simulink model "SSR_FIR"  (R2025a)
settings: Solver=VariableStepAuto  StartTime=0.0  StopTime=1000  RelTol=1e-3
InitFcn:
  | SSR=8;
  | TAPS=64;
  | Ts=1/SSR;
  | FCOEFF = fir1(TAPS-1,0.25);
undefined symbols (not defined in the file or in its folder): S, vsva2197, xcvc1902
libraries: hdlSSR x12, hdlBasic x6, hdlUtilities x3, dspsrcs4 x1, dspobslib x1, vmcUtilities x1
settings Model: Creator=catalinb  LastModifiedBy=robg
settings SolverCC: AlgebraicLoopSolver=TrustRegion
settings DebuggingCC: UnconnectedInputMsg=warning  UnconnectedOutputMsg=warning  UnconnectedLineMsg=warning
settings ModelReferenceCC: EnableRefExpFcnMdlSchedulingChecks=on
settings RTWCC: GPUComputeCapability=3.5  DLArmComputeVersion=19.05

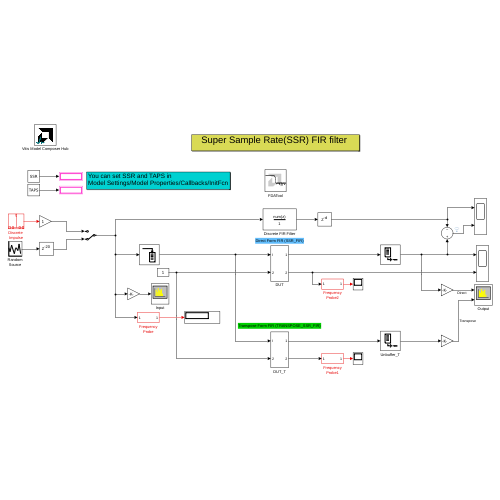
[thumbnail: Simulink's stored preview of the top-level diagram]
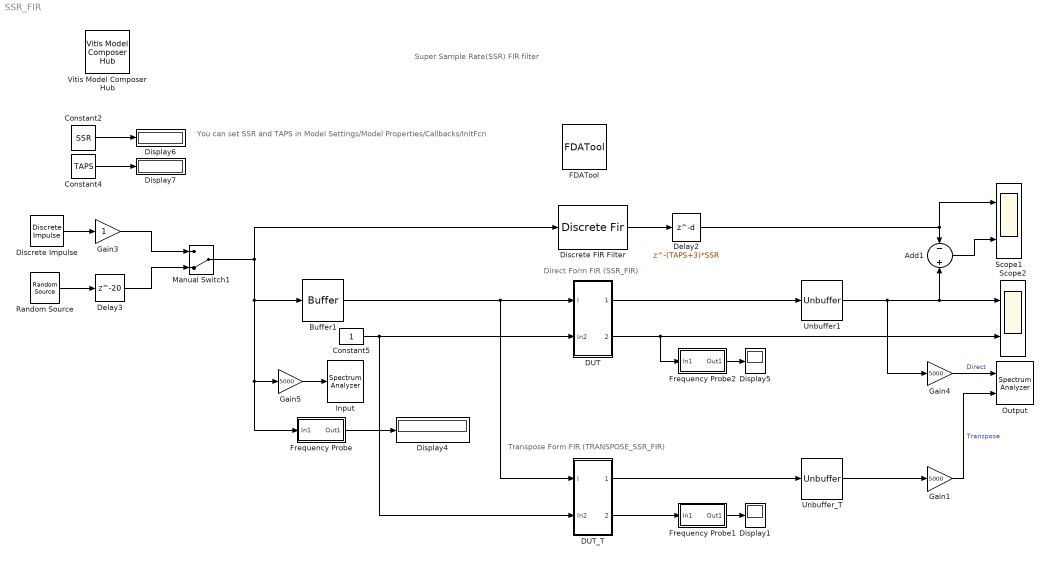
== system SSR_FIR ==
  note: You can set SSR and TAPS in
      | Model Settings/Model Properties/Callbacks/InitFcn
  note: Super Sample Rate(SSR) FIR filter
  note: Direct Form FIR (SSR_FIR)
  note: Transpose Form FIR (TRANSPOSE_SSR_FIR)
  Add1 : Sum  Inputs=-|+
  Buffer1 : Buffer  N=SSR  OutputFrames=off
  Constant2 : Constant  Value=SSR
  Constant4 : Constant  Value=TAPS
  Constant5 : Constant  SampleTime=-1
  DUT : Subsystem
  DUT_T : Subsystem
  Delay2 : Delay  DelayLength=(TAPS+3)*SSR
  Delay3 : Delay  DelayLength=20
  Discrete Impulse : dspsrcs4/Discrete  Impulse  SFcnStateName=COUNT  Delay=19  SampleTime=Ts  FrameSample=1  OutputFrames=off  dataType=double  isSigned=on  wordLen=16  udDataType=sfix(16)  fracBitsMode=Best precision  numFracBits=15  OutDataTypeStr=double  LastOutDataTypeStr=double
      settings: SFcnIsStateOwnerBlock=on
  Discrete FIR Filter : DiscreteFir  Coefficients=FCOEFF  InputProcessing=Columns as channels (frame based)
  Display{1,4..7} (5 alike) : Display
  FDATool : hdlUtilities/FDATool  block_type=fdatool
      settings: infoedit=FDATool
  Frequency Probe : Subsystem
  Frequency Probe1 : Subsystem
  Frequency Probe2 : Subsystem
  Gain1 : Gain  Gain=5000
  Gain3 : Gain
  Gain4 : Gain  Gain=5000
  Gain5 : Gain  Gain=5000
  Input : SpectrumAnalyzer  WindowPosition=[892.000000,252.000000,808.000000,450.000000,]  ScopeFrameLocation=window  SampleRate=5  AxesScaling=Manual  Span=8  StartFrequency=-4  StopFrequency=4  AveragingMethod=Exponential  YLimits=[35.8582 80.9757]  ChannelNames="[\"\"]"  AllowFFTLengthLessThanSamplesPerUpdate=on  DefaultConfigurationName=spbscopes.SpectrumAnalyzerBlockCfg
  Manual Switch1 : ManualSwitch  CurrentSetting=0
  Output : SpectrumAnalyzer  NumInputPorts=2  WindowPosition=[131.000000,278.000000,802.000000,452.000000,]  ScopeFrameLocation=window  SampleRate=5  AxesScaling=Manual  Span=8  StartFrequency=-4  StopFrequency=4  AveragingMethod=Exponential  YLimits=[-125.0298,37.1965]  ShowLegend=on  ChannelNames="[\"\"]"  AllowFFTLengthLessThanSamplesPerUpdate=on  DefaultConfigurationName=spbscopes.SpectrumAnalyzerBlockCfg
  Random Source : dspobslib/Random Source  SrcType=Uniform  NormMethod=Ziggurat  CltLength=12  MinVal=-1  MaxVal=1  MeanVal=0  VarVal=1  RepMode=Not repeatable  rawSeed=1  IsInherit=off  SampMode=Discrete  SampTime=Ts  SampFrame=1  DataType=Double  OutComplex=Real  OutputFrames=off
  Scope1 : Scope  NumInputPorts=2
      settings: ActiveDisplayYMinimum=-1.4468  ActiveDisplayYMaximum=1.4114  DataLoggingVariableName=ScopeData2
  Scope2 : Scope  NumInputPorts=2
      settings: ActiveDisplayYMinimum=-0.75312  ActiveDisplayYMaximum=0.71474
  Unbuffer1 : Unbuffer
  Unbuffer_T : Unbuffer
  Vitis Model Composer Hub : vmcUtilities/Vitis Model Composer Hub  Tag=genX  CodeGeneration=off  SubsystemName=DUT  BlockHierPath=SSR_FIR/DUT  CompilationType=HDLCompilation  SubsystemType=HDLNode  ExportTypeV2=IP Catalog  StartColumn=1  NumberOfColumns=1  TargetDirectory=./netlist  exportDesign=on  analyzeDesign=off  validateDesignOnHw=off  ExportType=AI Engines  IpVendor=xilinx.com  IpLibrary=hls  IpVersion=1.0  IpHWLanguage=Verilog  AieCompilerOptions={}  AieSimulatorOptions={}  CreateTestbench=off  TestbenchStackSize=10  RunRtlSim=off  RunCSim=off  RunAieSim=off  enableSimulationTimeout=on  enableGraphIterations=on  AieSimTimeout=50000  AieGraphIterations=-1  RunAieSimProfiling=off  LaunchVitisAnalyzer=off  PlotOutput=off  RunX86Sim=off  X86SimTimeout=10  GenHwImage=off  GenLibadfXo=on  GenHwValidationCode=off  PlatformType=Not Specified  HwSystemType=Baremetal  HwValidationTarget=hw  ProjDevice=xcvc1902-vsva2197-1LP-e-S  ProjDevicePart=xcvc1902-vsva2197-1LP-e-S  AIEType=AIE  SamplePeriod=-1  ClockFrequency=200  DataPathParallelism=1  xilinxfamily=versalaicore  part=xcvc1902  speed=-1LP-e-S  package=vsva2197  directory=./netlist/ip/DUT/src  testbench=off  incr_netlist=off  synthesis_tool=Vivado  clock_wrapper=Clock Enables  dbl_ovrd=According to Block Masks  dcm_input_clock_period=10  sysclk_period=10  simulink_period=1  eval_field=0  IPInfoJsonString="{\"DUTSubsystemName\":\"DUT\",\"HDLSubsystem\":{\"SubsystemName\":\"DUT\",\"IPName\":\"SSR_fir\",\"IPLibrary\":\"VMC\",\"IPVendor\":\"User Company\",\"IPVersion\":\"1.0\",\"TargetDirectory\":\"./netlist\",\"SubsystemDir\":\"./netlist/ip/DUT\",\"FreqHz\":\"100000000\"},\"SubsystemTag\":\"HDLNode\"}"  LogFileName=/proj/xhdhdstaff5/sdegala/Head1/HEAD/ModelComposer_Sept16/Vitis_Model_Composer/Examples/HDL/Digital_Filtering/SSR_FIR/netlist/model_composer.log  NThreads=4  IPConfigFile=/tmp/vmctmp-9769773316677438567/SSR_FIR_ipconfig.json
  wires:
  Gain3/1 -> Manual Switch1/1
  Unbuffer1/1 -> Gain4/1, Add1/2, Scope2/1
  Manual Switch1/1 -> Discrete FIR Filter/1, Buffer1/1, Frequency Probe/1(In1), Gain5/1
  Constant2/1 -> Display6/1
  Delay3/1 -> Manual Switch1/2
  Discrete Impulse/1 -> Gain3/1
  Frequency Probe2/1(Out1) -> Display5/1
  Gain4/1 -> Output/1  "Direct"
  Gain5/1 -> Input/1
  Delay2/1 -> Scope1/1, Add1/1
  DUT/1(Out1) -> Unbuffer1/1
  Buffer1/1 -> DUT/1(I), DUT_T/1(I)
  Constant5/1 -> DUT/2(In2), DUT_T/2(In2)
  Frequency Probe/1(Out1) -> Display4/1
  Add1/1 -> Scope1/2
  DUT/2(Out2) -> Scope2/2, Frequency Probe2/1(In1)
  Discrete FIR Filter/1 -> Delay2/1
  Constant4/1 -> Display7/1
  Random Source/1 -> Delay3/1
  DUT_T/1(Out1) -> Unbuffer_T/1
  Unbuffer_T/1 -> Gain1/1
  DUT_T/2(Out2) -> Frequency Probe1/1(In1)
  Gain1/1 -> Output/2  "Transpose"
  Frequency Probe1/1(Out1) -> Display1/1

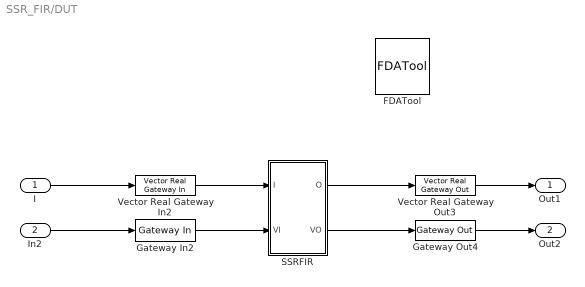
== system SSR_FIR/DUT ==
  I : Inport
  In2 : Inport  Port=2
  FDATool : hdlUtilities/FDATool  block_type=fdatool
      settings: infoedit=FDATool
  Gateway In2 : hdlBasic/Gateway In  gui_display_data_type=Boolean  arith_type=Boolean  n_bits=10  bin_pt=0  preci_type=Single  exp_width=8  frac_width=24  rows=1  columns=1  quantization="Round  (unbiased: +/- Inf)"  overflow=Saturate  period=1  UseAsADC=off  ADCChannel='1'  interface=None  automatic_assignment=on  address_offset=hex2dec('00')  intf_name=''  intf_description=''  default_value=0  timing_constraint=None  locs_specified=off  LOCs={}  io_standard={}  inherit_from_input=off  hdl_port=on  XmcBlockStatus=1  maskContainerNames=group4  block_type=gatewayin  block_config=sysgen:gateway_in_config  block_width_w=590  block_height_w=620  block_width=640  block_height=850
  Gateway Out4 : hdlBasic/Gateway Out  inherit_from_input=off  bool_to_boolean=off  hdl_port=on  rows=1  columns=1  UseAsDAC=off  DACChannel='1'  interface=None  automatic_assignment=on  address_offset=hex2dec('00')  intf_name=''  intf_description=''  timing_constraint=None  locs_specified=off  LOCs={}  io_standard={}  XmcBlockStatus=1  maskContainerNames=group4  block_type=gatewayout  block_config=sysgen:gateway_out_config  block_width_w=590  block_height_w=620  block_width=620  block_height=750
  SSRFIR : Subsystem  mask{OX=-1, OY=-1, DDR=on, SSR=SSR, TAPS=TAPS, COEFFICIENT=FCOEFF, I_HIGH=1, I_LOW=-16, C_HIGH=0, C_LOW=-17, O_HIGH=7, O_LOW=-16, ROUNDING=on, SYMMETRY="NS"}
      mask help:
      | OX, OY: Lower left coordinates of SSR*TAPS DSP48/DSP58 array; set to -1 to to turn off floorplanning
      |
      | DDR: Turn this on only if you are targetting Versal and clock speeds higher than 795/824/872MHz in the three speed grades; it will make timing closure possible but will use extra fabric resources; do not use this for 7-Series or UltraScale families
      |
      | COEFFICIENT: FIR coefficients, a vector of real values, separated by space or commas; only the first TAPS values are used
      |
      | I_HIGH,I_LOW: Input data fixed point range; if Model Composer fixed point data is Fix_m_n, m=I_HIGH-I_LOW+1 and n=-I_LOW
      |
      | C_HIGH,C_LOW: Coefficient fixed point range; the REAL COEFFICIENT values will be converted to fixed point using this range
      |
      | O_HIGH,O_LOW: Output data fixed point range; the internal sum of products will be truncated or rounded to this range
      |
      | ROUNDING: Will add 0.5 of output LSB before truncating the extra LSBs
      |
      | SYMMETRY: "NS" for non-symmetric, "ES" for even symmetric, "OS" for odd-symmetric; the filter order N will be TAPS, 2*TAPS and 2*TAPS-1 respectively
  Vector Real Gateway In2 : hdlSSR/Vector Real Gateway In  gui_display_data_type=Fixed-point  arith_type=Signed (2's comp)  n_bits=18  bin_pt=16  preci_type=Single  exp_width=8  frac_width=24  quantization="Round  (unbiased: +/- Inf)"  overflow=Saturate  period=1  sg_ssr=SSR  UseAsADC=off  ADCChannel='1'  interface=None  automatic_assignment=off  address_offset=hex2dec('00')  intf_name=''  intf_description=''  default_value=0  timing_constraint=None  locs_specified=off  LOCs={}  io_standard={}  inherit_from_input=off  hdl_port=on  interface_prev=1  block_type=realgatewayin_ssr  XmcBlockStatus=1  sg_ssr_prev=8  maskContainerNames=group4  block_width_w=590  block_height_w=670  block_width=640  block_height=850
      settings: SourceProductName=Xilinx SSR Blockset
  Vector Real Gateway Out3 : hdlSSR/Vector Real Gateway Out  inherit_from_input=off  hdl_port=on  sg_ssr=SSR  rows=1  columns=1  UseAsDAC=off  DACChannel='1'  interface=None  automatic_assignment=on  address_offset=hex2dec('00')  intf_name=''  intf_description=''  timing_constraint=None  locs_specified=off  LOCs={}  io_standard={}  block_type=realgatewayout_ssr  XmcBlockStatus=1  sg_ssr_prev=8  maskContainerNames=group4  block_width_w=590  block_height_w=620  block_width=620  block_height=750
      settings: SourceProductName=Xilinx SSR Blockset
  Out1 : Outport
  Out2 : Outport  Port=2
  wires:
  I/1 -> Vector Real Gateway In2/1
  Vector Real Gateway Out3/1 -> Out1/1
  SSRFIR/1(O) -> Vector Real Gateway Out3/1
  Gateway In2/1 -> SSRFIR/2(VI)
  Gateway Out4/1 -> Out2/1
  Vector Real Gateway In2/1 -> SSRFIR/1(I)
  In2/1 -> Gateway In2/1
  SSRFIR/2(VO) -> Gateway Out4/1

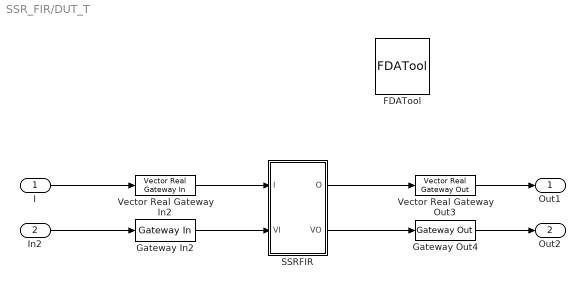
== system SSR_FIR/DUT_T ==
  I : Inport
  In2 : Inport  Port=2
  FDATool : hdlUtilities/FDATool  block_type=fdatool
      settings: infoedit=FDATool
  Gateway In2 : hdlBasic/Gateway In  gui_display_data_type=Boolean  arith_type=Boolean  n_bits=10  bin_pt=0  preci_type=Single  exp_width=8  frac_width=24  rows=1  columns=1  quantization="Round  (unbiased: +/- Inf)"  overflow=Saturate  period=1  UseAsADC=off  ADCChannel='1'  interface=None  automatic_assignment=on  address_offset=hex2dec('00')  intf_name=''  intf_description=''  default_value=0  timing_constraint=None  locs_specified=off  LOCs={}  io_standard={}  inherit_from_input=off  hdl_port=on  XmcBlockStatus=1  maskContainerNames=group4  block_type=gatewayin  block_config=sysgen:gateway_in_config  block_width_w=590  block_height_w=620  block_width=640  block_height=850
  Gateway Out4 : hdlBasic/Gateway Out  inherit_from_input=off  bool_to_boolean=off  hdl_port=on  rows=1  columns=1  UseAsDAC=off  DACChannel='1'  interface=None  automatic_assignment=on  address_offset=hex2dec('00')  intf_name=''  intf_description=''  timing_constraint=None  locs_specified=off  LOCs={}  io_standard={}  XmcBlockStatus=1  maskContainerNames=group4  block_type=gatewayout  block_config=sysgen:gateway_out_config  block_width_w=590  block_height_w=620  block_width=620  block_height=750
  SSRFIR : Subsystem  mask{OX=-1, OY=-1, DDR=on, SSR=SSR, TAPS=TAPS, COEFFICIENT=FCOEFF, I_HIGH=1, I_LOW=-16, C_HIGH=0, C_LOW=-17, O_HIGH=7, O_LOW=-16, ROUNDING=on, SYMMETRY="NS"}
      mask help:
      | OX, OY: Lower left coordinates of SSR*TAPS DSP48/DSP58 array; set to -1 to to turn off floorplanning
      |
      | DDR: Turn this on only if you are targetting Versal and clock speeds higher than 795/824/872MHz in the three speed grades; it will make timing closure possible but will use extra fabric resources; do not use this for 7-Series or UltraScale families
      |
      | COEFFICIENT: FIR coefficients, a vector of real values, separated by space or commas; only the first TAPS values are used
      |
      | I_HIGH,I_LOW: Input data fixed point range; if Model Composer fixed point data is Fix_m_n, m=I_HIGH-I_LOW+1 and n=-I_LOW
      |
      | C_HIGH,C_LOW: Coefficient fixed point range; the REAL COEFFICIENT values will be converted to fixed point using this range
      |
      | O_HIGH,O_LOW: Output data fixed point range; the internal sum of products will be truncated or rounded to this range
      |
      | ROUNDING: Will add 0.5 of output LSB before truncating the extra LSBs
      |
      | SYMMETRY: "NS" for non-symmetric, "ES" for even symmetric, "OS" for odd-symmetric; the filter order N will be TAPS, 2*TAPS and 2*TAPS-1 respectively
  Vector Real Gateway In2 : hdlSSR/Vector Real Gateway In  gui_display_data_type=Fixed-point  arith_type=Signed (2's comp)  n_bits=18  bin_pt=16  preci_type=Single  exp_width=8  frac_width=24  quantization="Round  (unbiased: +/- Inf)"  overflow=Saturate  period=1  sg_ssr=SSR  UseAsADC=off  ADCChannel='1'  interface=None  automatic_assignment=off  address_offset=hex2dec('00')  intf_name=''  intf_description=''  default_value=0  timing_constraint=None  locs_specified=off  LOCs={}  io_standard={}  inherit_from_input=off  hdl_port=on  interface_prev=1  block_type=realgatewayin_ssr  XmcBlockStatus=1  sg_ssr_prev=8  maskContainerNames=group4  block_width_w=590  block_height_w=670  block_width=640  block_height=850
      settings: SourceProductName=Xilinx SSR Blockset
  Vector Real Gateway Out3 : hdlSSR/Vector Real Gateway Out  inherit_from_input=off  hdl_port=on  sg_ssr=SSR  rows=1  columns=1  UseAsDAC=off  DACChannel='1'  interface=None  automatic_assignment=on  address_offset=hex2dec('00')  intf_name=''  intf_description=''  timing_constraint=None  locs_specified=off  LOCs={}  io_standard={}  block_type=realgatewayout_ssr  XmcBlockStatus=1  sg_ssr_prev=8  maskContainerNames=group4  block_width_w=590  block_height_w=620  block_width=620  block_height=750
      settings: SourceProductName=Xilinx SSR Blockset
  Out1 : Outport
  Out2 : Outport  Port=2
  wires:
  SSRFIR/2(VO) -> Gateway Out4/1
  In2/1 -> Gateway In2/1
  Vector Real Gateway In2/1 -> SSRFIR/1(I)
  Gateway Out4/1 -> Out2/1
  Gateway In2/1 -> SSRFIR/2(VI)
  SSRFIR/1(O) -> Vector Real Gateway Out3/1
  Vector Real Gateway Out3/1 -> Out1/1
  I/1 -> Vector Real Gateway In2/1

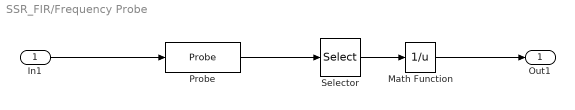
== system SSR_FIR/Frequency Probe ==
  In1 : Inport
  Math Function : Math  Operator=reciprocal
  Probe : Probe  ProbeWidth=off  ProbeComplexSignal=off
  Selector : Selector  InputPortWidth=2  IndexOptions=Index vector (dialog)  Indices=1  OutputSizes=1
  Out1 : Outport
  wires:
  Selector/1 -> Math Function/1
  Probe/1 -> Selector/1
  In1/1 -> Probe/1
  Math Function/1 -> Out1/1

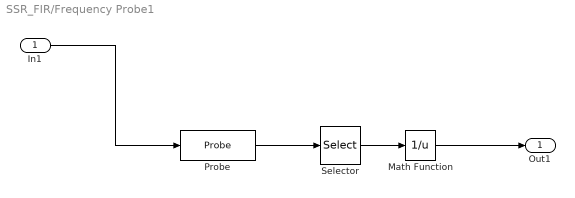
== system SSR_FIR/Frequency Probe1 ==
  In1 : Inport
  Math Function : Math  Operator=reciprocal
  Probe : Probe  ProbeWidth=off  ProbeComplexSignal=off
  Selector : Selector  InputPortWidth=2  IndexOptions=Index vector (dialog)  Indices=1  OutputSizes=1
  Out1 : Outport
  wires:
  Selector/1 -> Math Function/1
  Probe/1 -> Selector/1
  In1/1 -> Probe/1
  Math Function/1 -> Out1/1

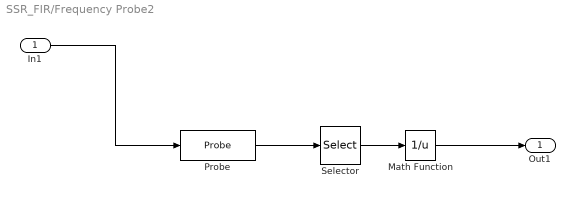
== system SSR_FIR/Frequency Probe2 ==
  In1 : Inport
  Math Function : Math  Operator=reciprocal
  Probe : Probe  ProbeWidth=off  ProbeComplexSignal=off
  Selector : Selector  InputPortWidth=2  IndexOptions=Index vector (dialog)  Indices=1  OutputSizes=1
  Out1 : Outport
  wires:
  Math Function/1 -> Out1/1
  In1/1 -> Probe/1
  Probe/1 -> Selector/1
  Selector/1 -> Math Function/1

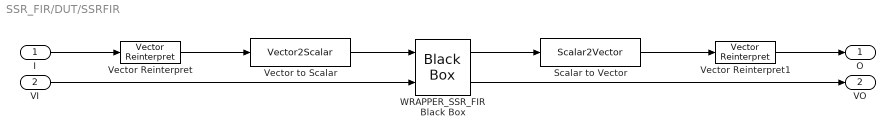
== system SSR_FIR/DUT/SSRFIR ==
  I : Inport
  VI : Inport  Port=2
  Scalar to Vector : hdlSSR/Scalar2Vector  Width=O_HIGH-O_LOW+1  sg_ssr=SSR  block_type=scalar2vector_ssr  XmcBlockStatus=1  sg_ssr_prev=8  maskContainerNames=group1
      settings: SourceProductName=Xilinx SSR Blockset
  Vector Reinterpret : hdlSSR/Vector Reinterpret  force_arith_type=on  arith_type=Unsigned  force_bin_pt=on  bin_pt=0  sg_ssr=SSR  block_type=reinterpret_ssr  XmcBlockStatus=1  sg_ssr_prev=8  maskContainerNames=group1
      settings: SourceProductName=Xilinx SSR Blockset
  Vector Reinterpret1 : hdlSSR/Vector Reinterpret  force_arith_type=on  arith_type="Signed  (2's comp)"  force_bin_pt=on  bin_pt=-O_LOW  sg_ssr=SSR  block_type=reinterpret_ssr  XmcBlockStatus=1  sg_ssr_prev=8  maskContainerNames=group1
      settings: SourceProductName=Xilinx SSR Blockset
  Vector to Scalar : hdlSSR/Vector2Scalar  sg_ssr=SSR  block_type=vector2scalar_ssr  XmcBlockStatus=1  sg_ssr_prev=8  maskContainerNames=group1
      settings: SourceProductName=Xilinx SSR Blockset
  WRAPPER_SSR_FIR Black Box : hdlBasic/Black Box  init_code=WRAPPER_SSR_FIR_config  sim_method=Vivado Simulator  engine_block=ModelSim  verbose=on  XmcBlockStatus=1  maskContainerNames=group1  block_type=blackbox2  block_config=sysgen:black_box_config
  O : Outport
  VO : Outport  Port=2
  wires:
  WRAPPER_SSR_FIR Black Box/2 -> VO/1
  WRAPPER_SSR_FIR Black Box/1 -> Scalar to Vector/1
  Vector Reinterpret1/1 -> O/1
  Vector Reinterpret/1 -> Vector to Scalar/1
  I/1 -> Vector Reinterpret/1
  VI/1 -> WRAPPER_SSR_FIR Black Box/2
  Vector to Scalar/1 -> WRAPPER_SSR_FIR Black Box/1
  Scalar to Vector/1 -> Vector Reinterpret1/1

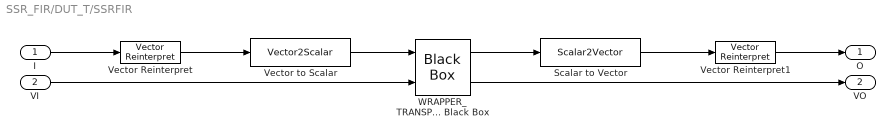
== system SSR_FIR/DUT_T/SSRFIR ==
  I : Inport
  VI : Inport  Port=2
  Scalar to Vector : hdlSSR/Scalar2Vector  Width=O_HIGH-O_LOW+1  sg_ssr=SSR  block_type=scalar2vector_ssr  XmcBlockStatus=1  sg_ssr_prev=8  maskContainerNames=group1
      settings: SourceProductName=Xilinx SSR Blockset
  Vector Reinterpret : hdlSSR/Vector Reinterpret  force_arith_type=on  arith_type=Unsigned  force_bin_pt=on  bin_pt=0  sg_ssr=SSR  block_type=reinterpret_ssr  XmcBlockStatus=1  sg_ssr_prev=8  maskContainerNames=group1
      settings: SourceProductName=Xilinx SSR Blockset
  Vector Reinterpret1 : hdlSSR/Vector Reinterpret  force_arith_type=on  arith_type="Signed  (2's comp)"  force_bin_pt=on  bin_pt=-O_LOW  sg_ssr=SSR  block_type=reinterpret_ssr  XmcBlockStatus=1  sg_ssr_prev=8  maskContainerNames=group1
      settings: SourceProductName=Xilinx SSR Blockset
  Vector to Scalar : hdlSSR/Vector2Scalar  sg_ssr=SSR  block_type=vector2scalar_ssr  XmcBlockStatus=1  sg_ssr_prev=8  maskContainerNames=group1
      settings: SourceProductName=Xilinx SSR Blockset
  WRAPPER_TRANSPOSE_SSR_FIR Black Box : hdlBasic/Black Box  init_code=WRAPPER_TRANSPOSE_SSR_FIR_config  sim_method=Vivado Simulator  engine_block=ModelSim  verbose=on  XmcBlockStatus=1  maskContainerNames=group1  block_type=blackbox2  block_config=sysgen:black_box_config
  O : Outport
  VO : Outport  Port=2
  wires:
  Scalar to Vector/1 -> Vector Reinterpret1/1
  Vector to Scalar/1 -> WRAPPER_TRANSPOSE_SSR_FIR Black Box/1
  VI/1 -> WRAPPER_TRANSPOSE_SSR_FIR Black Box/2
  I/1 -> Vector Reinterpret/1
  Vector Reinterpret/1 -> Vector to Scalar/1
  Vector Reinterpret1/1 -> O/1
  WRAPPER_TRANSPOSE_SSR_FIR Black Box/1 -> Scalar to Vector/1
  WRAPPER_TRANSPOSE_SSR_FIR Black Box/2 -> VO/1
